simulink model "d_mixvf_sim"  (R2022b)
settings: Solver=FixedStepAuto  StartTime=0.0  StopTime=5.0  FixedStep=0.01  RelTol=1e-3
StopFcn:
  | %d_mixvf_plot
model workspace (MAT data in the model file):
  initial_position = [3 2.8]
settings Model: Creator=p282037  LastModifiedBy=lukas
settings SolverCC: AlgebraicLoopSolver=TrustRegion
settings DataIOCC: ReturnWorkspaceOutputs=off
settings OptimizationCC: LifeSpan=inf
settings DebuggingCC: UnconnectedInputMsg=warning  UnconnectedOutputMsg=warning  UnconnectedLineMsg=warning  SFExecutionAtInitializationDiag=none  SFMachineParentedDataDiag=warning  ArithmeticOperatorsInVariantConditions=warning
settings ModelReferenceCC: EnableRefExpFcnMdlSchedulingChecks=on
settings SFSimCC: SimUseLocalCustomCode=off  CustomCodeUndefinedFunction=UseInterfaceOnly
settings RTWCC: RTWUseLocalCustomCode=off
settings CodeAppCC: StateflowObjectComments=on

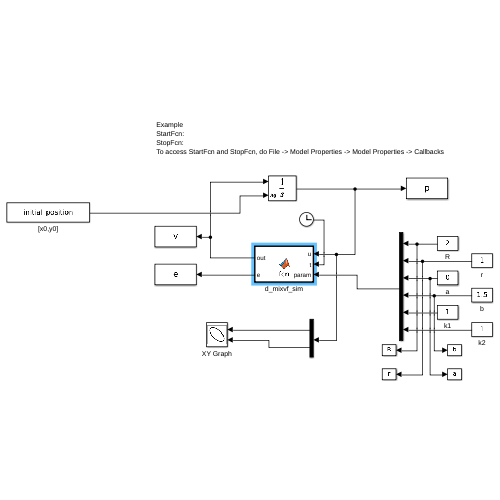
[thumbnail: Simulink's stored preview of the top-level diagram]
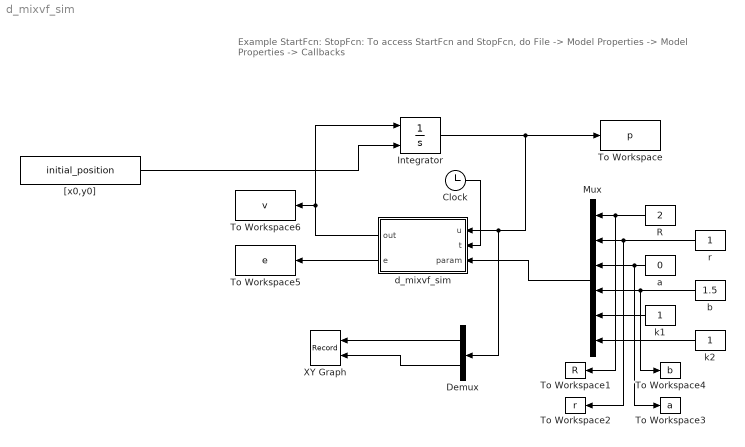
== system d_mixvf_sim ==
  note: Example
      | StartFcn:
      | StopFcn:
      | To access StartFcn and StopFcn, do File -> Model Properties -> Model Properties -> Callbacks
  Clock : Clock
  Demux : Demux  Outputs=2
  Integrator : Integrator  InitialConditionSource=external  InitialCondition=[0 0.5 3]
  Mux : Mux  Inputs=6
  R : Constant  Value=2
  To Workspace : ToWorkspace  VariableName=p  SampleTime=-1
      settings: Save2DSignal=2-D array (concatenate along first dimension)
  To Workspace1 : ToWorkspace  VariableName=R  SampleTime=-1
      settings: MaxDataPoints=1
  To Workspace2 : ToWorkspace  VariableName=r  SampleTime=-1
      settings: MaxDataPoints=1
  To Workspace3 : ToWorkspace  VariableName=a  SampleTime=-1
      settings: MaxDataPoints=1
  To Workspace4 : ToWorkspace  VariableName=b  SampleTime=-1
      settings: MaxDataPoints=1
  To Workspace5 : ToWorkspace  VariableName=e  SaveFormat=Timeseries  SampleTime=-1
  To Workspace6 : ToWorkspace  VariableName=v  SaveFormat=Timeseries  SampleTime=-1
  XY Graph : Record  FileSettingsInternal="{\"entries\":[{\"content\":{\"excelSettings\":{\"content\":{},\"type\":\"Streamout.ExcelSettings\"}},\"type\":\"Streamout.FileSettingStorage\",\"uuid\":\"7bbd014f-18f8-4bd0-8de6-029c92e9f613\"}],\"packageUris\":[\"http://schema.mathworks.com/mf0/streamout_blocks/R2020a\"],\"version\":\"1.0\"}"  Layout=[1 1]  SignalsInternal="{\"entries\":[{\"content\":{\"signals\":[{\"content\":{\"blockPath\":[\"d_mixvf_sim/XY Graph\"],\"channel\":[],\"dimensions\":[1],\"domain\":\"d_mixvf_sim/XY Graph\",\"lineColor\":\"#a2142f\",\"plots\":[1],\"port\":1,\"sid\":[\"\"],\"signalID\":83246,\"signalName\":\"Demux:1\"},\"type\":\"RecordBlkView.Signal\",\"uuid\":\"c98c5642-9dfb-4531-9f4e-a407fe7d5419\"},{\"content\":{\"blockPath\":[\"d_mixvf_sim/XY Graph\"],\"channel\":[],\"dimensions\":[1],\"domain\":\"d_mixvf_sim/XY Graph\",\"lineColor\":\"#139fff\",\"plots\":[1],\"port\":2,\"sid\":[\"\"],\"signalID\":83250,\"signalName\":\"Demux:2\"},\"type\":\"RecordBlkView.Signal\",\"uuid\":\"4cee8184-29cc-4bbb-8df6-8adcb37f48a1\"}]},\"type\":\"RecordBlkView.InputSignals\",\"uuid\":\"dd7f1e3a-69df-4a7d-883d-d061a3e1c433\"}],\"packageUris\":[\"http://schema.mathworks.com/mf0/streamout_blocks/R2020a\"],\"version\":\"1.0\"}"  VisualizationBindings="{\"xyplotplugin\":{\"info\":[{\"series\":[{\"bindingParametersList\":[{\"parameter\":\"X-Axis\",\"signalID\":83246,\"signalName\":\"Demux:1\"},{\"parameter\":\"Y-Axis\",\"signalID\":83250,\"signalName\":\"Demux:2\"}],\"seriesID\":30884}],\"subplotID\":1}]}}"  CompatibilityTag=XY  st=-1
  "[x0,y0]" : Constant  Value=initial_position
  a : Constant  Value=0
  b : Constant  Value=1.5
  d_mixvf_sim : MATLAB Function  TreatAsAtomicUnit=on
  k1 : Constant
  k2 : Constant
  r : Constant
  wires:
  d_mixvf_sim/1(out) -> To Workspace6/1, Integrator/1
  r/1 -> To Workspace2/1, Mux/2
  a/1 -> To Workspace3/1, Mux/3
  b/1 -> To Workspace4/1, Mux/4
  R/1 -> To Workspace1/1, Mux/1
  Mux/1 -> d_mixvf_sim/3(param)
  d_mixvf_sim/2(e) -> To Workspace5/1
  k1/1 -> Mux/5
  k2/1 -> Mux/6
  Demux/1 -> XY Graph/1
  Demux/2 -> XY Graph/2
  Clock/1 -> d_mixvf_sim/2(t)
  Integrator/1 -> Demux/1, d_mixvf_sim/1(u), To Workspace/1
  "[x0,y0]"/1 -> Integrator/2

== matlab function d_mixvf_sim/d_mixvf_sim ==
  data: u input; t input; out output; param input; e output
function [out,e] = fcn(u, t, param)

x=u(1); y=u(2);
R=param(1); R=param(2); a=param(3); b=param(4); k1=param(5); k=param(6);
e=zeros(2,1);

%% 
E = [0, -1; 1, 0];
R = 2; beta = pi/4;

k1 = 1;
phi = x^2 + y^2 - R^2;
grad = [2*x; 2*y];
vfphi = E*grad - k1*phi*grad;
    
a = 1; b = 0.5;
k = 1;

vphi1 = x^2/a^2 + (y+R)^2/b^2 - 1;
grad = [2*x/a^2; 2*(y+R)/b^2];
vfvphi1 = E*grad - k*vphi1*grad;

vphi2 = ((x-R)*cos(beta)+y*sin(beta))^2/a^2 + ((x-R)*sin(beta)-y*cos(beta))^2/b^2 - 1;
grad = [2^(1/2)*((2^(1/2)*y)/2 + (2^(1/2)*(x - 2))/2) - 4*2^(1/2)*((2^(1/2)*y)/2 - (2^(1/2)*(x - 2))/2); 
     4*2^(1/2)*((2^(1/2)*y)/2 - (2^(1/2)*(x - 2))/2) + 2^(1/2)*((2^(1/2)*y)/2 + (2^(1/2)*(x - 2))/2)];
vfvphi2 = E*grad - k*vphi2*grad;

vphi3 = (x+2.6)^2/b^2 + y^2/a^2 - 1;
grad = [8*x + 104/5; 2*y];
vfvphi3 = E*grad - k*vphi3*grad;

vphi4 = (x+1.4)^2/b^2 + y^2/a^2 - 1;
grad = [8*x + 56/5; 2*y];
vfvphi4 = E*grad - k*vphi4*grad;

vphi5 = ((x-0.9)^2+(y-R)^2)*((x+0.9)^2+(y-R)^2) - 0.9;
grad = [(2*x - 9/5)*((x + 9/10)^2 + (y - 2)^2) + (2*x + 9/5)*((x - 9/10)^2 + (y - 2)^2); 
         (2*y - 4)*((x - 9/10)^2 + (y - 2)^2) + (2*y - 4)*((x + 9/10)^2 + (y - 2)^2)];
vfvphi5 = E*grad - k*vphi5*grad;

%% new; journal version;
c1 = -0.72; c2 = -0.72; c3 = -0.2; c4 = -0.2; c5 = -0.23;
l1 = 0.1; l2 = 0.1;

%%% zero-inside bump function
if( vphi1 <= c1 )
    kq1 = 0;
else
    if( vphi1 < 0 )
        f1 = exp( l1/(c1 - vphi1) );
        f2 = exp( l2/(vphi1 - 0) );
        kq1 = f1/(f1+f2);
    else
        kq1 = 1;
    end
end

if( vphi2 < c2 )
    kq2 = 0;
else
    if( vphi2 < 0 )
        f1 = exp( l1/(c2 - vphi2) );
        f2 = exp( l2/(vphi2 - 0) );
        kq2 = f1/(f1+f2);
    else
        kq2 = 1;
    end    
end

if( vphi3 < c3 )
    kq3 = 0;
else
    if( vphi3 < 0 )
        f1 = exp( l1/(c3 - vphi3) );
        f2 = exp( l2/(vphi3 - 0) );
        kq3 = f1/(f1+f2);
    else
        kq3 = 1;
    end
end

if( vphi4 < c4 )
    kq4 = 0;
else
    if( vphi4 < 0 )
        f1 = exp( l1/(c4 - vphi4) );
        f2 = exp( l2/(vphi4 - 0) );
        kq4 = f1/(f1+f2);
    else
        kq4 = 1;
    end
end

if( vphi5 < c5 )
    kq5 = 0;
else
    if( vphi5 < 0 )
        f1 = exp( l1/(c5 - vphi5) );
        f2 = exp( l2/(vphi5 - 0) );
        kq5 = f1/(f1+f2);
    else
        kq5 = 1;
    end
end

%%% zero-outside bump function
kr1 = 1-kq1;
kr2 = 1-kq2;
kr3 = 1-kq3;
kr4 = 1-kq4;
kr5 = 1-kq5;


%%% composite vector field
v = kq1*kq2*kq3*kq4*kq5 * vfphi / norm(vfphi) + ...
    kr1 * vfvphi1 / norm(vfvphi1) + ...
    kr2 * vfvphi2 / norm(vfvphi2) + ...
    kr3 * vfvphi3 / norm(vfvphi3) + ...
    kr4 * vfvphi4 / norm(vfvphi4) + ...
    kr5 * vfvphi5 / norm(vfvphi5);
      

out=v;
e=[phi; vphi1];
